simulink model "ContinSoftStart_55kWt_done_v20_discrete"  (R2019b)
settings: Solver=ode23t  StartTime=0.0  StopTime=10  MaxStep=1e-3  RelTol=1e-6  EnableMultiTasking=on
undefined symbols (not defined in the file): f, J, L1sig, L2sig, P2n, ph_deg, r1, r2, Ts, Vm
libraries: powerlib x20, simulink x3
settings Model: Creator=NPT  LastModifiedBy=NPT
settings DataIOCC: LimitDataPoints=on  SaveFormat=Array  ReturnWorkspaceOutputs=off
settings OptimizationCC: LifeSpan=inf
settings DebuggingCC: SolverPrmCheckMsg=warning  SFUnexpectedBacktrackingDiag=warning  SFNoUnconditionalDefaultTransitionDiag=warning  SFExecutionAtInitializationDiag=none  ArithmeticOperatorsInVariantConditions=warning
settings HardwareCC: ProdBitPerPointer=32  ProdBitPerSizeT=32  ProdBitPerPtrDiffT=32  ProdLargestAtomicFloat=None  ProdIntDivRoundTo=Undefined  ProdEndianess=Unspecified  ProdWordSize=32  ProdHWDeviceType=32-bit Generic
settings ModelReferenceCC: PropagateSignalLabelsOutOfModel=off
settings SFSimCC: SimUseLocalCustomCode=off  CustomCodeUndefinedFunction=UseInterfaceOnly
settings RTWCC: RTWUseLocalCustomCode=off
settings CodeAppCC: StateflowObjectComments=on
settings GRTTargetCC: TargetLangStandard=C89/C90 (ANSI)  GeneratePreprocessorConditionals=Disable all
settings ConfigComp: CovMetricSettings=dw  CovHtmlReporting=on  CovSaveCumulativeToWorkspaceVar=on  CovSaveSingleToWorkspaceVar=on  CovExternalEMLEnable=off  CovSFcnEnable=off
settings SimscapeCC: SimscapeNormalizeSystem=off

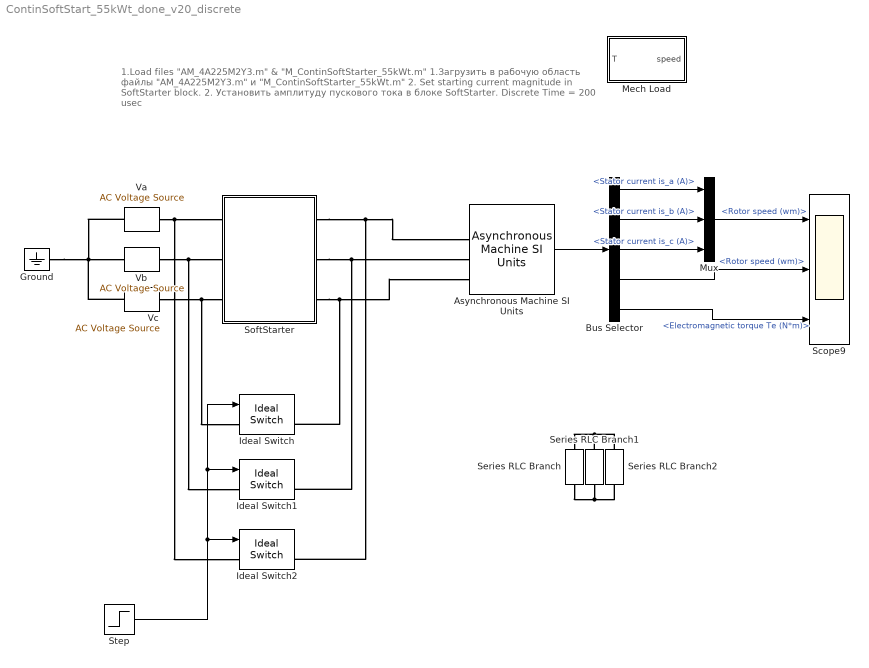
== system ContinSoftStart_55kWt_done_v20_discrete ==
  note: 1.Load files "AM_4A225M2Y3.m" & "M_ContinSoftStarter_55kWt.m"
      | 1.Загрузить в рабочую область файлы "AM_4A225M2Y3.m" и "M_ContinSoftStarter_55kWt.m"
      |
      | 2. Set starting current magnitude in SoftStarter block.
      | 2. Установить амплитуду пускового тока в блоке SoftStarter.
      |
      |
      | Discrete Time = 200 usec
  Asynchronous Machine SI Units : powerlib/Machines/Asynchronous Machine SI Units  RotorType=Squirrel-cage  PresetModel=No  MechanicalLoad=Torque Tm  ShowDetailedParameters=on  ReferenceFrame=Rotor  Units=SI  MeasurementBus=off  NominalParameters=[P2n 380 50]  Stator=[r1 L1sig]  Rotor=[r2 L2sig]  Cage1=[ 0.022 0.226/377]  Cage2=[ 0.022 0.226/377]  Lm=L0  Mechanical=[J 0 1]  PolePairs=2  InitialConditions=[1 0 0 0 0 0 0 0]  SimulateSaturation=off  Saturation=[14.03593122, 27.81365428, 53.79336849, 72.68890987, 97.98006896, 148.6815601, 215.7428561, 302.9841135, 420.4778367 ; 230, 322, 414, 460, 506, 552, 598, 644, 690]  LoadFlowParameters=1492000  TsPowergui=0  TsBlock=-1  IterativeModel=Trapezoidal non iterative  IterativeDiscreteModel=Trapezoidal non iterative  Pmec=10000
      settings: SourceProductName=Simscape Electrical
  Bus Selector : BusSelector  OutputSignals=Stator measurements.Stator current is_a (A),Stator measurements.Stator current is_b (A),Stator measurements.Stator current is_c (A),Mechanical.Rotor speed (wm),Mechanical.Electromagnetic torque Te (N*m)
  Ground : powerlib/Elements/Ground  LConnTagsString=a
      settings: SourceProductName=Simscape Electrical
  Ideal Switch : powerlib/Power Electronics/Ideal Switch  Ron=0.001  Lon=0  IC=0  Rs=1e5  Cs=inf  Measurements=on
      settings: SourceProductName=Simscape Electrical
  Ideal Switch1 : powerlib/Power Electronics/Ideal Switch  Ron=0.001  Lon=0  IC=0  Rs=1e5  Cs=inf  Measurements=on
      settings: SourceProductName=Simscape Electrical
  Ideal Switch2 : powerlib/Power Electronics/Ideal Switch  Ron=0.001  Lon=0  IC=0  Rs=1e5  Cs=inf  Measurements=on
      settings: SourceProductName=Simscape Electrical
  Mech Load : Subsystem
  Mux : Mux  Inputs=3
  Scope9 : Scope  NumInputPorts=3
  Series RLC Branch : powerlib/Elements/Series RLC Branch  LConnTagsString=__new0  RConnTagsString=__new0  BranchType=RL  Resistance=1  Inductance=1e-3  SetiL0=off  InitialCurrent=0  Capacitance=1e-6  Setx0=off  InitialVoltage=0  Measurements=None
      settings: SourceProductName=Simscape Electrical
  Series RLC Branch1 : powerlib/Elements/Series RLC Branch  LConnTagsString=__new0  RConnTagsString=__new0  BranchType=RL  Resistance=1  Inductance=1e-3  SetiL0=off  InitialCurrent=0  Capacitance=1e-6  Setx0=off  InitialVoltage=0  Measurements=None
      settings: SourceProductName=Simscape Electrical
  Series RLC Branch2 : powerlib/Elements/Series RLC Branch  LConnTagsString=__new0  RConnTagsString=__new0  BranchType=RL  Resistance=1  Inductance=1e-3  SetiL0=off  InitialCurrent=0  Capacitance=1e-6  Setx0=off  InitialVoltage=0  Measurements=None
      settings: SourceProductName=Simscape Electrical
  SoftStarter : Subsystem
  Step : Step  Time=3.5  SampleTime=0
  Va : powerlib/Electrical Sources/AC Voltage Source  Amplitude=Vm  Phase=ph_deg(1)  Frequency=f  SampleTime=-1  Measurements=None  BusType=swing  Pref=10e3  Qref=0  Qmin=-inf  Qmax=+inf
      settings: SourceProductName=Simscape Electrical
  Vb : powerlib/Electrical Sources/AC Voltage Source  Amplitude=Vm  Phase=ph_deg(2)  Frequency=f  SampleTime=-1  Measurements=None  BusType=swing  Pref=10e3  Qref=0  Qmin=-inf  Qmax=+inf
      settings: SourceProductName=Simscape Electrical
  Vc : powerlib/Electrical Sources/AC Voltage Source  Amplitude=Vm  Phase=ph_deg(3)  Frequency=f  SampleTime=-1  Measurements=None  BusType=swing  Pref=10e3  Qref=0  Qmin=-inf  Qmax=+inf
      settings: SourceProductName=Simscape Electrical
  wires:
  Asynchronous Machine SI Units/1 -> Bus Selector/1
  Bus Selector/3 -> Mux/3  "<Stator current is_c (A)>"
  Bus Selector/2 -> Mux/2  "<Stator current is_b (A)>"
  Bus Selector/1 -> Mux/1  "<Stator current is_a (A)>"
  Bus Selector/4 -> Scope9/2  "<Rotor speed (wm)>"
  Bus Selector/5 -> Scope9/3  "<Electromagnetic torque Te (N*m)>"
  Mux/1 -> Scope9/1  "<Rotor speed (wm)>"
  Step/1 -> Ideal Switch/1, Ideal Switch1/1, Ideal Switch2/1
  connections:
  Ground/LConn1 -- Vb/LConn1 -- Va/LConn1 -- Vc/LConn1
  Vc/RConn1 -- Ideal Switch/LConn1 -- SoftStarter/LConn3
  Series RLC Branch/RConn1 -- Series RLC Branch1/RConn1 -- Series RLC Branch2/RConn1
  Series RLC Branch2/LConn1 -- Series RLC Branch1/LConn1 -- Series RLC Branch/LConn1
  SoftStarter/RConn2 -- Ideal Switch1/RConn1 -- Asynchronous Machine SI Units/LConn2
  SoftStarter/RConn1 -- Ideal Switch2/RConn1 -- Asynchronous Machine SI Units/LConn1
  SoftStarter/RConn3 -- Ideal Switch/RConn1 -- Asynchronous Machine SI Units/LConn3
  Vb/RConn1 -- Ideal Switch1/LConn1 -- SoftStarter/LConn2
  Va/RConn1 -- Ideal Switch2/LConn1 -- SoftStarter/LConn1

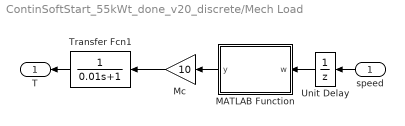
== system ContinSoftStart_55kWt_done_v20_discrete/Mech Load ==
  speed : Inport
  MATLAB Function : MATLAB Function  TreatAsAtomicUnit=on
  Mc : Gain  Gain=10
  Transfer Fcn1 : TransferFcn  Denominator=[0.01 1]
  Unit Delay : UnitDelay  SampleTime=-1  HasFrameUpgradeWarning=on
  T : Outport
  wires:
  MATLAB Function/1(y) -> Mc/1
  Unit Delay/1 -> MATLAB Function/1(w)
  Mc/1 -> Transfer Fcn1/1
  Transfer Fcn1/1 -> T/1
  speed/1 -> Unit Delay/1

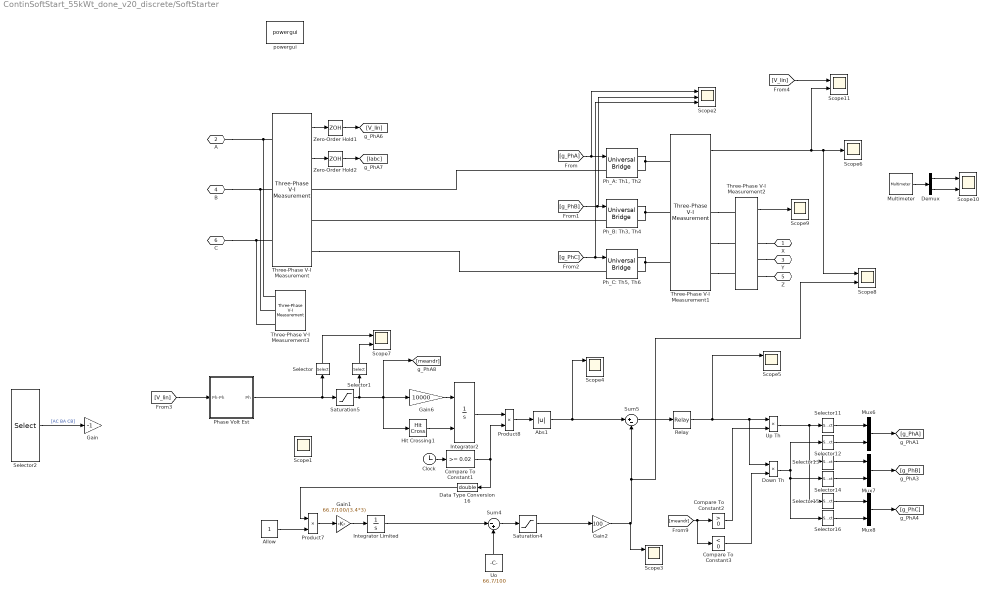
== system ContinSoftStart_55kWt_done_v20_discrete/SoftStarter ==
  Abs1 : Abs
  Allow : Constant
  Clock : Clock
  Compare To Constant1 : simulink/Logic and Bit Operations/Compare To Constant  relop=>=  const=0.02  OutDataTypeStr=boolean
  Compare To Constant2 : simulink/Logic and Bit Operations/Compare To Constant  relop=>  const=0  OutDataTypeStr=uint8
  Compare To Constant3 : simulink/Logic and Bit Operations/Compare To Constant  relop=<  const=0  OutDataTypeStr=uint8
  Data Type Conversion16 : DataTypeConversion  OutDataTypeStr=double
  Demux : Demux  Outputs=2
  Down Th : Product
  Gain : Gain  Gain=-1
  Gain1 : Gain  Gain=66.7/100/(3.4*3)
  Gain2 : Gain  Gain=100
  Gain6 : Gain  Gain=10000
  Hit Crossing1 : HitCross
  Integrator Limited : Integrator  LimitOutput=on  UpperSaturationLimit=66.7/100  LowerSaturationLimit=0
  Integrator2 : Integrator  ExternalReset=either  LimitOutput=on  UpperSaturationLimit=100  LowerSaturationLimit=-100
  Multimeter : powerlib/Measurements/Multimeter  PhasorSimulation=off  OutputType=Complex  sel=[1 4]  L=5  Gain=[1 1]  yselected={'Usw1: SoftStarter/Ph_A: Th1, Th2','Isw1: SoftStarter/Ph_A: Th1, Th2'};  PSBOutputType=1  PSBequivalent=0  AxesSetting=[0,0.1,-100,100]  Display=0  SavedBlockNames=-11
      settings: SourceProductName=Simscape Electrical
  Mux6 : Mux  Inputs=2
  Mux7 : Mux  Inputs=2
  Mux8 : Mux  Inputs=2
  "Ph_A: Th1, Th2" : powerlib/Power Electronics/Universal Bridge  Arms=1  SnubberResistance=1e5  SnubberCapacitance=inf  Device=Thyristors  Ron=1e-3  Lon=0  ForwardVoltages="[  0  0  ]"  ForwardVoltage=0  GTOparameters=[ 10e-6 , 20e-6 ]  IGBTparameters=[ 1e-6 , 2e-6 ]  Measurements=All voltages and currents  Measurements_2=None  converterType=Rectifier
      settings: SourceProductName=Simscape Electrical
  "Ph_B: Th3, Th4 " : powerlib/Power Electronics/Universal Bridge  Arms=1  SnubberResistance=1e5  SnubberCapacitance=inf  Device=Thyristors  Ron=1e-3  Lon=0  ForwardVoltages="[  0  0  ]"  ForwardVoltage=0  GTOparameters=[ 10e-6 , 20e-6 ]  IGBTparameters=[ 1e-6 , 2e-6 ]  Measurements=None  Measurements_2=None  converterType=Rectifier
      settings: SourceProductName=Simscape Electrical
  "Ph_C: Th5, Th6" : powerlib/Power Electronics/Universal Bridge  Arms=1  SnubberResistance=1e5  SnubberCapacitance=inf  Device=Thyristors  Ron=1e-3  Lon=0  ForwardVoltages="[  0  0  ]"  ForwardVoltage=0  GTOparameters=[ 10e-6 , 20e-6 ]  IGBTparameters=[ 1e-6 , 2e-6 ]  Measurements=None  Measurements_2=None  converterType=Rectifier
      settings: SourceProductName=Simscape Electrical
  Phase Volt Est : Subsystem
  Product7 : Product
  Product8 : Product  OutDataTypeStr=double
  Relay : Relay
  Saturation4 : Saturate  UpperLimit=66.7/100  LowerLimit=2.8/100
  Saturation5 : Saturate  UpperLimit=1  LowerLimit=-1
  Scope{1,7..8,10..11} (5 alike) : Scope  NumInputPorts=2
  Scope{2..5} (4 alike) : Scope  NumInputPorts=3
  Scope6 : Scope
  Scope9 : Scope
  Selector{,1,13..14} (4 alike) : Selector  InputPortWidth=3  IndexOptions=Index vector (dialog)  Indices=[2]  OutputSizes=1
  Selector11 : Selector  InputPortWidth=3  IndexOptions=Index vector (dialog)  Indices=[1]  OutputSizes=1
  Selector12 : Selector  InputPortWidth=3  IndexOptions=Index vector (dialog)  Indices=[1]  OutputSizes=1
  Selector15 : Selector  InputPortWidth=3  IndexOptions=Index vector (dialog)  Indices=[3]  OutputSizes=1
  Selector16 : Selector  InputPortWidth=3  IndexOptions=Index vector (dialog)  Indices=[3]  OutputSizes=1
  Selector2 : Selector  InputPortWidth=3  IndexOptions=Index vector (dialog)  Indices=[3 1 2]  OutputSizes=1
  Sum4 : Sum  Inputs=|-+
  Sum5 : Sum  Inputs=|+-
  Three-Phase V-I Measurement : powerlib/Measurements/Three-Phase V-I Measurement  VoltageMeasurement=phase-to-phase  SetLabelV=off  LabelV=Vabc  Vpu=off  VpuLL=off  CurrentMeasurement=yes  SetLabelI=off  LabelI=Iabc  Ipu=off  Pbase=100e6  Vbase=500e3  OutputType=Complex  PhasorSimulation=off  PSBequivalent=0
      settings: SourceProductName=Simscape Electrical
  Three-Phase V-I Measurement1 : powerlib/Measurements/Three-Phase V-I Measurement  VoltageMeasurement=phase-to-phase  SetLabelV=off  LabelV=Vabc  Vpu=off  VpuLL=off  CurrentMeasurement=yes  SetLabelI=off  LabelI=Iabc  Ipu=off  Pbase=100e6  Vbase=500e3  OutputType=Complex  PhasorSimulation=off  PSBequivalent=0
      settings: SourceProductName=Simscape Electrical
  Three-Phase V-I Measurement2 : powerlib/Measurements/Three-Phase V-I Measurement  VoltageMeasurement=phase-to-ground  SetLabelV=off  LabelV=Vabc  Vpu=off  VpuLL=off  CurrentMeasurement=yes  SetLabelI=off  LabelI=Iabc  Ipu=off  Pbase=100e6  Vbase=500e3  OutputType=Complex  PhasorSimulation=off  PSBequivalent=0
      settings: SourceProductName=Simscape Electrical
  Three-Phase V-I Measurement3 : powerlib/Measurements/Three-Phase V-I Measurement  VoltageMeasurement=phase-to-ground  SetLabelV=off  LabelV=Vabc  Vpu=off  VpuLL=off  CurrentMeasurement=yes  SetLabelI=off  LabelI=Iabc  Ipu=off  Pbase=100e6  Vbase=500e3  OutputType=Complex  PhasorSimulation=off  PSBequivalent=0
      settings: SourceProductName=Simscape Electrical
  Uo : Constant  Value=66.7/100
  Up Th : Product
  Zero-Order Hold1 : ZeroOrderHold  SampleTime=2e-4
  Zero-Order Hold2 : ZeroOrderHold  SampleTime=2e-4
  powergui : powerlib/powergui  Priority=1  SimulationMode=Continuous  SampleTime=Ts  frequency=60  Iterations=50  frequencyindice=50  Pbase=100e6  ErrMax=1e-4  UnitsV=kV  UnitsW=MW  buscounter=0  FunctionMessages=off  echomessages=off  EnableUseOfTLC=off  CurrentSourceSwitches=on  DisableSnubberDevices=off  DisableRonSwitches=off  DisableVfSwitches=off  DisplayEquations=off  AutomaticDiscreteSolvers=off  SolverType=Tustin  Interpol=off  ExternalGateDelay=off  methode=off  Ts=0  x0status=zero  SPID=off  SwTol=0  HookPort=off  NonlinearTolerance=1e-4  nMaxIteration=100  ContinueOnMaxIteration=off  RestoreLinks=warning  ResistiveCurrentMeasurement=off  Frange=[0:2:500]  Ylog=off  Xlog=on  ShowGrid=off  save=off  variable=ZData  structure=0  ZoomFFT=off  StartTime=0.0  cycles=1  DisplayStyle=1  fundamental=60  FreqAxis=off  MaxFrequency=1000  frequencyindicesteady=1  RmsSteady=1  display=off
      settings: SourceProductName=Simscape Electrical
  X : PMIOPort  Side=Right
  A : PMIOPort  Port=2  Side=Left
  Y : PMIOPort  Port=3  Side=Right
  B : PMIOPort  Port=4  Side=Left
  Z : PMIOPort  Port=5  Side=Right
  C : PMIOPort  Port=6  Side=Left
  wires:
  Three-Phase V-I Measurement/2 -> Zero-Order Hold2/1
  Three-Phase V-I Measurement/1 -> Zero-Order Hold1/1
  Sum4/1 -> Saturation4/1
  [g_PhA] -> Scope2/1, "Ph_A: Th1, Th2"/1
  [g_PhB] -> Scope2/2, "Ph_B: Th3, Th4 "/1
  [g_PhC] -> Scope2/3, "Ph_C: Th5, Th6"/1
  Allow/1 -> Product7/2
  Uo/1 -> Sum4/2
  Phase Volt Est/1(Ph) -> Selector/1, Saturation5/1
  Gain6/1 -> Integrator2/1
  Saturation5/1 -> [meandr], Hit Crossing1/1, Gain6/1, Selector1/1
  Hit Crossing1/1 -> Integrator2/2
  Clock/1 -> Compare To Constant1/1
  Integrator2/1 -> Product8/1
  Compare To Constant1/1 -> Data Type Conversion16/1, Product8/2
  Product8/1 -> Abs1/1
  Saturation4/1 -> Gain2/1
  Sum5/1 -> Relay/1
  [meandr] -> Compare To Constant3/1, Compare To Constant2/1
  Relay/1 -> Scope5/1, Down Th/1, Up Th/1
  Compare To Constant2/1 -> Up Th/2
  Compare To Constant3/1 -> Down Th/2
  Up Th/1 -> Selector13/1, Selector15/1, Selector11/1
  Selector11/1 -> Mux6/1
  Down Th/1 -> Selector14/1, Selector16/1, Selector12/1
  Selector12/1 -> Mux6/2
  Selector14/1 -> Mux7/2
  Selector13/1 -> Mux7/1
  Selector16/1 -> Mux8/2
  Selector15/1 -> Mux8/1
  Data Type Conversion16/1 -> Product7/1
  Mux6/1 -> [g_PhA]
  Mux7/1 -> [g_PhB]
  Mux8/1 -> [g_PhC]
  Zero-Order Hold1/1 -> [V_lin]
  Zero-Order Hold2/1 -> [Iabc]
  Abs1/1 -> Scope4/1, Sum5/1
  Product7/1 -> Gain1/1
  Gain1/1 -> Integrator Limited/1
  Integrator Limited/1 -> Sum4/1
  [V_lin] -> Phase Volt Est/1(Ph-Ph)
  Three-Phase V-I Measurement1/1 -> Scope11/2, Scope8/1, Scope6/1
  Selector/1 -> Scope7/1
  Selector1/1 -> Scope7/2
  Three-Phase V-I Measurement2/1 -> Scope9/1
  Gain2/1 -> Scope3/1, Scope8/2, Sum5/2
  Multimeter/1 -> Demux/1
  Demux/1 -> Scope10/1
  Demux/2 -> Scope10/2
  Selector2/1 -> Gain/1  "[AC BA CB]"
  [V_lin] -> Scope11/1
  connections:
  C/RConn1 -- Three-Phase V-I Measurement3/LConn3 -- Three-Phase V-I Measurement/LConn3
  B/RConn1 -- Three-Phase V-I Measurement3/LConn2 -- Three-Phase V-I Measurement/LConn2
  A/RConn1 -- Three-Phase V-I Measurement3/LConn1 -- Three-Phase V-I Measurement/LConn1
  Three-Phase V-I Measurement/RConn3 -- "Ph_C: Th5, Th6"/LConn1
  "Ph_A: Th1, Th2"/LConn1 -- Three-Phase V-I Measurement/RConn1
  "Ph_C: Th5, Th6"/RConn1 -- "Ph_C: Th5, Th6"/RConn2 -- Three-Phase V-I Measurement1/LConn3
  "Ph_B: Th3, Th4 "/RConn1 -- "Ph_B: Th3, Th4 "/RConn2 -- Three-Phase V-I Measurement1/LConn2
  "Ph_A: Th1, Th2"/RConn1 -- Three-Phase V-I Measurement1/LConn1 -- "Ph_A: Th1, Th2"/RConn2
  "Ph_B: Th3, Th4 "/LConn1 -- Three-Phase V-I Measurement/RConn2
  Three-Phase V-I Measurement1/RConn2 -- Three-Phase V-I Measurement2/LConn2
  Three-Phase V-I Measurement1/RConn1 -- Three-Phase V-I Measurement2/LConn1
  Three-Phase V-I Measurement1/RConn3 -- Three-Phase V-I Measurement2/LConn3
  Three-Phase V-I Measurement2/RConn1 -- X/RConn1
  Three-Phase V-I Measurement2/RConn2 -- Y/RConn1
  Three-Phase V-I Measurement2/RConn3 -- Z/RConn1

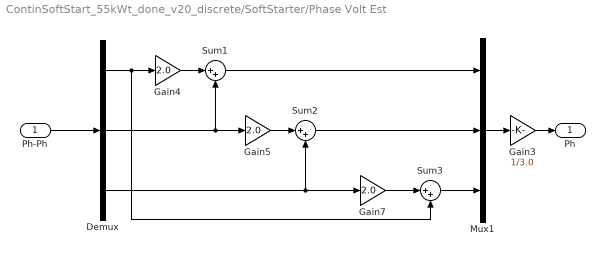
== system ContinSoftStart_55kWt_done_v20_discrete/SoftStarter/Phase Volt Est ==
  Ph-Ph : Inport
  Demux : Demux  Outputs=3
  Gain3 : Gain  Gain=1/3.0
  Gain4 : Gain  Gain=2.0
  Gain5 : Gain  Gain=2.0
  Gain7 : Gain  Gain=2.0
  Mux1 : Mux  Inputs=3
  Sum1 : Sum  Inputs=|++
  Sum2 : Sum  Inputs=|++
  Sum3 : Sum  Inputs=|++
  Ph : Outport
  wires:
  Demux/2 -> Gain5/1, Sum1/2
  Gain5/1 -> Sum2/1
  Sum2/1 -> Mux1/2
  Gain4/1 -> Sum1/1
  Gain7/1 -> Sum3/1
  Sum1/1 -> Mux1/1
  Sum3/1 -> Mux1/3
  Demux/1 -> Sum3/2, Gain4/1
  Ph-Ph/1 -> Demux/1
  Mux1/1 -> Gain3/1
  Demux/3 -> Gain7/1, Sum2/2
  Gain3/1 -> Ph/1

== matlab function ContinSoftStart_55kWt_done_v20_discrete/Mech Load/MATLAB Function ==
  data: w input; y output
function y = fcn(w)
%#codegen

if w > 0.01
    temp = 1;
elseif w < -0.01
    temp = -1;
else
    temp = 0;  
end

y = temp;
